simulink model "system_integration_v2"  (R2024a)
settings: Solver=FixedStepDiscrete  StartTime=0.0  StopTime=2  RelTol=1e-3
values from neighbouring files (symbols this model uses):
  Ts = 1/Fs    (= 7.50007500075e-06)    [new_generation_coeff.m]    (also in simon_test.m; simple_fft_test.m = 1/F; testPSD_c2d.m; testPSD_simulink.m)
undefined symbols (not defined in the file or in its folder): magnitude
libraries: hdlsllib x84, embmathops x6, hdlmdlgenlib x1, dsphdlxfrm2 x1
(part 2 of 5)

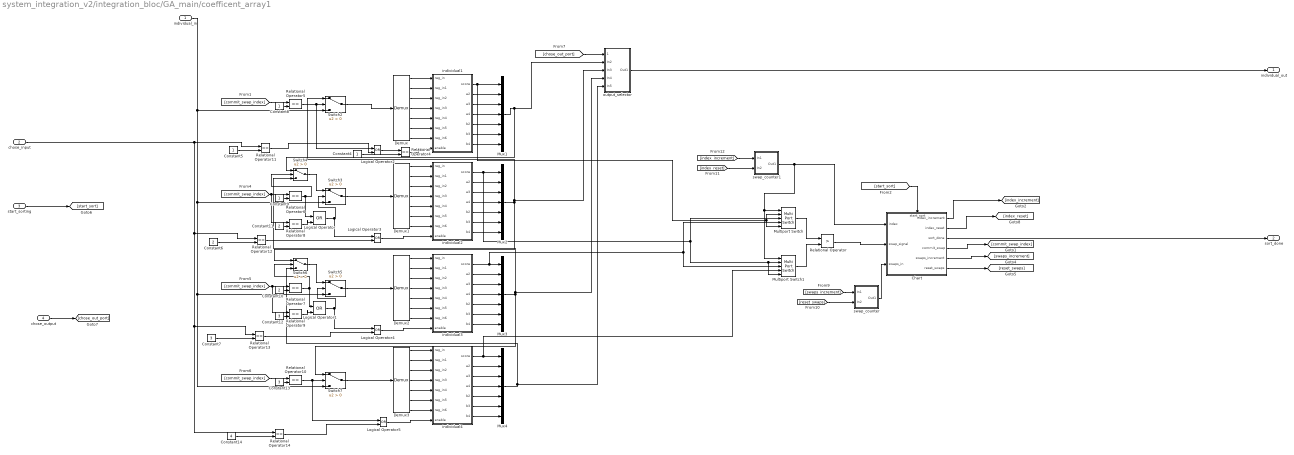
== system system_integration_v2/integration_bloc/GA_main/coefficent_array1 ==
  individual_in : Inport
  chose_input : Inport  Port=2
  start_sorting : Inport  Port=3
  chose_output : Inport  Port=4
  Chart : Stateflow chart  TreatAsAtomicUnit=on
      settings: PortSchema="{\"entries\":[{\"content\":{\"sides\":[{\"content\":{\"connectorIds\":[\"In1\",\"In4\",\"In3\"]},\"type\":\"ConnectorPlacement.EquallySpacedRectSide\",\"uuid\":\"bd2dafac-a5a9-4836-b8bd-cefb36fb6626\"},{\"content\":{\"connectorIds\":[\"Out1\",\"Out2\",\"Out3\",\"Out4\",\"Out5\",\"Out6\"],\"side\":\"RIGHT\"},\"type\":\"ConnectorPlacement.EquallySpacedRectSide\",\"uuid\":\"b2eb894e-8d56-4038-acbe-51c43d919a15\"},{\"content\":{\"connectorIds\":[\"In2\"],\"side\":\"TOP\"},\"type\":\"ConnectorPlacement.EquallySpacedRectSide\",\"uuid\":\"645ecb99-1eca-4a2d-8e44-d34ac75e3d1a\"}]},\"type\":\"ConnectorPlacement.EquallySpacedConnector\",\"uuid\":\"63f53eab-c5ec-482c-b992-d953653b0c27\"}],\"packageUris\":[\"http://schema.mathworks.com/mf0/Connector/R2020b\"],\"version\":\"1.0\"}"
  Constant10 : Constant  Value=2  OutDataTypeStr=fixdt(0,4,0)  SampleTime=Ts
  Constant11 : Constant  Value=2  OutDataTypeStr=fixdt(0,4,0)  SampleTime=Ts
  Constant12 : Constant  Value=3  OutDataTypeStr=fixdt(0,4,0)  SampleTime=Ts
  Constant13 : Constant  Value=3  OutDataTypeStr=fixdt(0,4,0)  SampleTime=Ts
  Constant14 : Constant  Value=4  OutDataTypeStr=fixdt(0,4,0)  SampleTime=Ts
  Constant{4..5,8..9} (4 alike) : Constant  OutDataTypeStr=fixdt(0,4,0)  SampleTime=Ts
  Constant6 : Constant  Value=2  OutDataTypeStr=fixdt(0,4,0)  SampleTime=Ts
  Constant7 : Constant  Value=3  OutDataTypeStr=fixdt(0,4,0)  SampleTime=Ts
  Demux{,1..3} (4 alike) : Demux  Outputs=7
  Logical Operator{,1..5} (6 alike) : Logic  Operator=OR  IconShape=distinctive  AllPortsSameDT=off  OutDataTypeStr=boolean
  Multiport Switch : MultiPortSwitch  DataPortForDefault=Additional data port  DiagnosticForDefault=None  SaturateOnIntegerOverflow=off  InputSameDT=off
  Multiport Switch1 : MultiPortSwitch  DataPortForDefault=Additional data port  DiagnosticForDefault=None  SaturateOnIntegerOverflow=off  InputSameDT=off
  Mux{1..4} (4 alike) : Mux  Inputs=7
  Relational Operator : RelationalOperator  Operator=>  OutDataTypeStr=boolean  InputSameDT=off
  Relational Operator{4..14} (11 alike) : RelationalOperator  Operator===  OutDataTypeStr=boolean  RndMeth=Simplest  InputSameDT=off
  Switch{2..7} (6 alike) : Switch  Criteria=u2 > Threshold  SaturateOnIntegerOverflow=off  InputSameDT=off
  individual1 : Subsystem
  individual2 : Subsystem
  individual3 : Subsystem
  individual4 : Subsystem
  output_selector : Subsystem
  swap_counter : Subsystem
  swap_counter1 : Subsystem
  individual_out : Outport  OutDataTypeStr=fixdt(1,64,32)
  sort_done : Outport  Port=2
  wires:
  individual4/7(b4) -> Mux4/7
  individual4/6(b3) -> Mux4/6
  individual4/5(b2) -> Mux4/5
  individual4/4(a4) -> Mux4/4
  individual4/3(a3) -> Mux4/3
  individual4/2(a2) -> Mux4/2
  Demux3/7 -> individual4/7(reg_in6)
  Demux3/6 -> individual4/6(reg_in5)
  Demux3/5 -> individual4/5(reg_in4)
  Demux3/4 -> individual4/4(reg_in3)
  Demux3/3 -> individual4/3(reg_in2)
  Demux3/2 -> individual4/2(reg_in1)
  Demux3/1 -> individual4/1(reg_in)
  individual3/7(b4) -> Mux3/7
  individual3/6(b3) -> Mux3/6
  individual3/5(b2) -> Mux3/5
  individual3/4(a4) -> Mux3/4
  individual3/3(a3) -> Mux3/3
  individual3/2(a2) -> Mux3/2
  Demux2/7 -> individual3/7(reg_in6)
  Demux2/6 -> individual3/6(reg_in5)
  Demux2/5 -> individual3/5(reg_in4)
  Demux2/4 -> individual3/4(reg_in3)
  Demux2/3 -> individual3/3(reg_in2)
  Demux2/2 -> individual3/2(reg_in1)
  Demux2/1 -> individual3/1(reg_in)
  Demux1/6 -> individual2/6(reg_in5)
  Demux1/5 -> individual2/5(reg_in4)
  Demux1/4 -> individual2/4(reg_in3)
  Demux1/3 -> individual2/3(reg_in2)
  Demux1/2 -> individual2/2(reg_in1)
  Demux1/1 -> individual2/1(reg_in)
  Demux1/7 -> individual2/7(reg_in6)
  individual2/7(b4) -> Mux2/7
  individual2/6(b3) -> Mux2/6
  individual2/5(b2) -> Mux2/5
  individual2/4(a4) -> Mux2/4
  individual1/7(b4) -> Mux1/7
  Demux/7 -> individual1/7(reg_in6)
  Mux4/1 -> output_selector/5(In5), Switch6/3
  Chart/2(index_reset) -> [index_reset]
  [index_reset] -> swap_counter1/2(In2)
  [index_increment] -> swap_counter1/1(In1)
  Constant14/1 -> Relational Operator14/2
  Relational Operator14/1 -> Logical Operator5/2
  Relational Operator13/1 -> Logical Operator4/2
  Constant7/1 -> Relational Operator13/2
  Relational Operator12/1 -> Logical Operator3/2
  Constant6/1 -> Relational Operator12/2
  Relational Operator11/1 -> Logical Operator2/2
  Constant5/1 -> Relational Operator11/2
  chose_output/1 -> [chose_out_port]
  Chart/3(sort_done) -> sort_done/1
  [start_sort] -> Chart/2(start_sort)
  individual2/3(a3) -> Mux2/3
  individual1/4(a4) -> Mux1/4
  Demux/4 -> individual1/4(reg_in3)
  individual1/2(a2) -> Mux1/2
  Relational Operator4/1 -> individual1/8(enable)
  individual1/6(b3) -> Mux1/6
  Demux/2 -> individual1/2(reg_in1)
  individual1/5(b2) -> Mux1/5
  Logical Operator2/1 -> Relational Operator4/1
  Constant10/1 -> Relational Operator7/2
  Relational Operator9/1 -> Logical Operator1/2
  Switch2/1 -> Demux/1
  Multiport Switch1/1 -> Relational Operator/2
  Relational Operator7/1 -> Switch6/2, Logical Operator1/1
  individual2/2(a2) -> Mux2/2
  Switch5/1 -> Demux2/1
  Chart/1(index_increment) -> [index_increment]
  Switch7/1 -> Demux3/1
  Constant8/1 -> Relational Operator5/2
  individual3/1(score) -> Multiport Switch/4, Multiport Switch1/3, Mux3/1
  Mux2/1 -> Switch6/1, Switch2/1, output_selector/3(In3)
  Demux/3 -> individual1/3(reg_in2)
  Logical Operator4/1 -> individual3/8(enable)
  Relational Operator/1 -> Chart/4(swap_signal)
  chose_input/1 -> Relational Operator11/1, Relational Operator12/1, Relational Operator13/1, Relational Operator14/1
  Demux/6 -> individual1/6(reg_in5)
  [chose_out_port] -> output_selector/1(chose_port)
  individual2/1(score) -> Multiport Switch1/2, Multiport Switch1/5, Multiport Switch/3, Mux2/1
  output_selector/1(Out1) -> individual_out/1
  Switch6/1 -> Switch5/1
  [commit_swap_index] -> Relational Operator10/1
  Constant12/1 -> Relational Operator9/2
  Constant13/1 -> Relational Operator10/2
  Constant4/1 -> Relational Operator4/2
  Relational Operator6/1 -> Switch4/2, Logical Operator/1
  individual4/1(score) -> Mux4/1, Multiport Switch1/4
  Switch3/1 -> Demux1/1
  individual_in/1 -> Switch2/3, Switch3/3, Switch5/3, Switch7/3
  Demux/5 -> individual1/5(reg_in4)
  Logical Operator/1 -> Switch3/2, Logical Operator3/1
  Chart/4(commit_swap) -> [commit_swap_index]
  start_sorting/1 -> [start_sort]
  Constant11/1 -> Relational Operator8/2
  Multiport Switch/1 -> Relational Operator/1
  Logical Operator5/1 -> individual4/8(enable)
  Logical Operator3/1 -> individual2/8(enable)
  [commit_swap_index] -> Relational Operator7/1, Relational Operator9/1
  [commit_swap_index] -> Relational Operator6/1, Relational Operator8/1
  Relational Operator8/1 -> Logical Operator/2
  Chart/6(reset_swaps) -> [reset_swaps]
  Mux1/1 -> output_selector/2(In2), Switch4/1
  [commit_swap_index] -> Relational Operator5/1
  [swaps_increment] -> swap_counter/1(In1)
  Relational Operator5/1 -> Switch2/2, Logical Operator2/1
  individual1/3(a3) -> Mux1/3
  swap_counter/1(Out1) -> Chart/3(swaps_in)
  [reset_swaps] -> swap_counter/2(In2)
  Relational Operator10/1 -> Switch7/2, Logical Operator5/1
  Mux3/1 -> Switch7/1, Switch4/3, output_selector/4(In4)
  Demux/1 -> individual1/1(reg_in)
  individual1/1(score) -> Multiport Switch/2, Multiport Switch/5, Mux1/1
  Switch4/1 -> Switch3/1
  swap_counter1/1(Out1) -> Chart/1(index), Multiport Switch/1, Multiport Switch1/1
  Chart/5(swaps_increment) -> [swaps_increment]
  Constant9/1 -> Relational Operator6/2
  Logical Operator1/1 -> Switch5/2, Logical Operator4/1

== system system_integration_v2/integration_bloc/GA_main/generation_counter ==
  In1 : Inport
  In2 : Inport  Port=2
  Add : Sum  OutDataTypeStr=fixdt(0,16,0)  AccumDataTypeStr=fixdt(0,16,0)
  Constant18 : Constant  OutDataTypeStr=fixdt(0,16,0)  SampleTime=Ts
  Constant19 : Constant  Value=0  OutDataTypeStr=fixdt(0,16,0)  SampleTime=Ts
  Constant20 : Constant  Value=0  OutDataTypeStr=fixdt(0,16,0)  SampleTime=Ts
  Delay : Delay  DelayLength=1  InitialCondition=0  SampleTime=Ts
  Switch : Switch  Criteria=u2 > Threshold  OutDataTypeStr=fixdt(0,16,0)  SaturateOnIntegerOverflow=off  InputSameDT=off
  Switch8 : Switch  Criteria=u2 > Threshold  OutDataTypeStr=fixdt(0,16,0)  SaturateOnIntegerOverflow=off  InputSameDT=off
  Out1 : Outport
  wires:
  Constant19/1 -> Switch/3
  Switch8/1 -> Add/2
  Switch/1 -> Add/1
  Delay/1 -> Out1/1, Switch8/3
  In2/1 -> Switch8/2
  Add/1 -> Delay/1
  Constant20/1 -> Switch8/1
  Constant18/1 -> Switch/1
  In1/1 -> Switch/2

== system system_integration_v2/integration_bloc/GA_main/index_counter ==
  In1 : Inport
  In2 : Inport  Port=2
  Add : Sum  OutDataTypeStr=fixdt(0,4,0)  AccumDataTypeStr=fixdt(0,4,0)
  Constant18 : Constant  OutDataTypeStr=fixdt(0,4,0)  SampleTime=Ts
  Constant19 : Constant  Value=0  OutDataTypeStr=fixdt(0,4,0)  SampleTime=Ts
  Constant20 : Constant  Value=0  OutDataTypeStr=fixdt(0,4,0)  SampleTime=Ts
  Delay : Delay  DelayLength=1  InitialCondition=0  SampleTime=Ts
  Switch : Switch  Criteria=u2 > Threshold  OutDataTypeStr=fixdt(0,4,0)  SaturateOnIntegerOverflow=off  InputSameDT=off
  Switch8 : Switch  Criteria=u2 > Threshold  OutDataTypeStr=fixdt(0,4,0)  SaturateOnIntegerOverflow=off  InputSameDT=off
  index_counter : Outport
  wires:
  Constant19/1 -> Switch/3
  Switch8/1 -> Add/2
  Switch/1 -> Add/1
  Delay/1 -> index_counter/1, Switch8/3
  In2/1 -> Switch8/2
  Add/1 -> Delay/1
  Constant20/1 -> Switch8/1
  Constant18/1 -> Switch/1
  In1/1 -> Switch/2

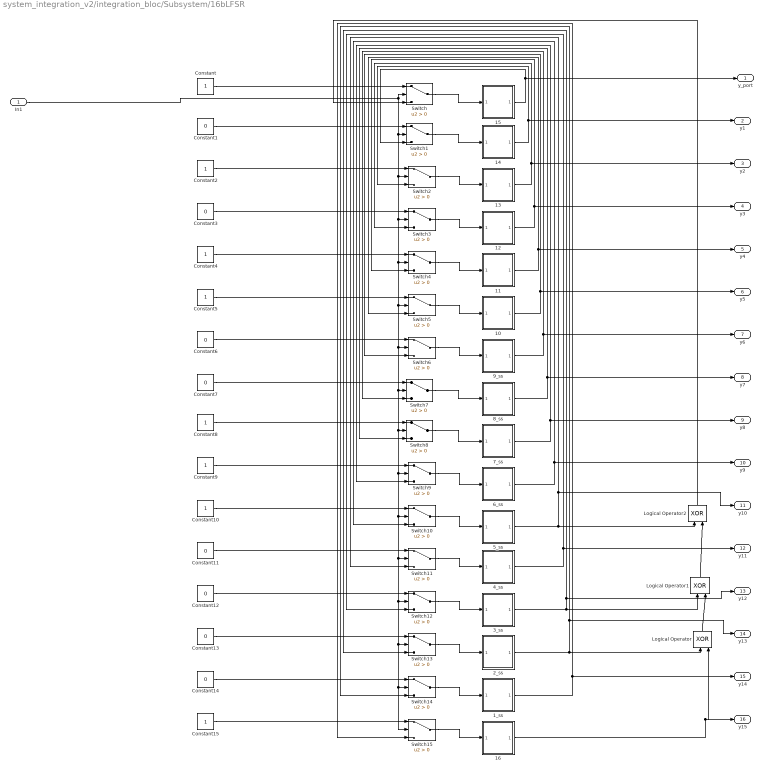
== system system_integration_v2/integration_bloc/Subsystem/16bLFSR ==
  In1 : Inport
  10 : Subsystem
  11 : Subsystem
  12 : Subsystem
  13 : Subsystem
  14 : Subsystem
  15 : Subsystem
  16 : Subsystem
  1_ss : Subsystem
  2_ss : Subsystem
  3_ss : Subsystem
  4_ss : Subsystem
  5_ss : Subsystem
  6_ss : Subsystem
  7_ss : Subsystem
  8_ss : Subsystem
  9_ss : Subsystem
  Constant{,2,4..5,8..10,15} (8 alike) : Constant  OutDataTypeStr=boolean  SampleTime=Ts
  Constant{1,3,6..7,11..14} (8 alike) : Constant  Value=0  OutDataTypeStr=boolean  SampleTime=Ts
  Logical Operator : Logic  Operator=XOR  IconShape=distinctive  AllPortsSameDT=off  OutDataTypeStr=boolean
  Logical Operator1 : Logic  Operator=XOR  IconShape=distinctive  AllPortsSameDT=off  OutDataTypeStr=boolean
  Logical Operator2 : Logic  Operator=XOR  IconShape=distinctive  AllPortsSameDT=off  OutDataTypeStr=boolean
  Switch{,1..15} (16 alike) : Switch  Criteria=u2 > Threshold  SaturateOnIntegerOverflow=off  InputSameDT=off
  y_port : Outport
  y1 : Outport  Port=2
  y2 : Outport  Port=3
  y3 : Outport  Port=4
  y4 : Outport  Port=5
  y5 : Outport  Port=6
  y6 : Outport  Port=7
  y7 : Outport  Port=8
  y8 : Outport  Port=9
  y9 : Outport  Port=10
  y10 : Outport  Port=11
  y11 : Outport  Port=12
  y12 : Outport  Port=13
  y13 : Outport  Port=14
  y14 : Outport  Port=15
  y15 : Outport  Port=16
  wires:
  5_ss/1(reg_out) -> Logical Operator2/1, y10/1, Switch11/3
  6_ss/1(reg_out) -> y9/1, Switch10/3
  2_ss/1(reg_out) -> Logical Operator/1, y13/1, Switch14/3
  11/1(reg_out) -> y4/1, Switch5/3
  Logical Operator2/1 -> Switch/3
  Constant13/1 -> Switch13/1
  Switch13/1 -> 2_ss/1(reg_in)
  3_ss/1(reg_out) -> Logical Operator1/1, y12/1, Switch13/3
  4_ss/1(reg_out) -> y11/1, Switch12/3
  Constant/1 -> Switch/1
  Constant4/1 -> Switch4/1
  Constant2/1 -> Switch2/1
  In1/1 -> Switch/2, Switch15/2, Switch14/2, Switch13/2, Switch12/2, Switch11/2, Switch10/2, Switch9/2, Switch8/2, Switch7/2, Switch6/2, Switch5/2, Switch4/2, Switch3/2, Switch2/2, Switch1/2
  Switch12/1 -> 3_ss/1(reg_in)
  15/1(reg_out) -> y_port/1, Switch1/3
  Switch1/1 -> 14/1(reg_in)
  Constant8/1 -> Switch8/1
  Constant6/1 -> Switch6/1
  Constant5/1 -> Switch5/1
  Constant14/1 -> Switch14/1
  Constant11/1 -> Switch11/1
  Switch5/1 -> 10/1(reg_in)
  Constant9/1 -> Switch9/1
  Logical Operator/1 -> Logical Operator1/2
  Switch2/1 -> 13/1(reg_in)
  7_ss/1(reg_out) -> y8/1, Switch9/3
  Logical Operator1/1 -> Logical Operator2/2
  Switch11/1 -> 4_ss/1(reg_in)
  Constant7/1 -> Switch7/1
  Switch6/1 -> 9_ss/1(reg_in)
  Switch/1 -> 15/1(reg_in)
  Constant12/1 -> Switch12/1
  Switch4/1 -> 11/1(reg_in)
  Constant15/1 -> Switch15/1
  16/1(reg_out) -> y15/1, Logical Operator/2
  13/1(reg_out) -> y2/1, Switch3/3
  Switch9/1 -> 6_ss/1(reg_in)
  Switch7/1 -> 8_ss/1(reg_in)
  Constant10/1 -> Switch10/1
  Switch14/1 -> 1_ss/1(reg_in)
  Switch3/1 -> 12/1(reg_in)
  Switch15/1 -> 16/1(reg_in)
  9_ss/1(reg_out) -> y6/1, Switch7/3
  Constant3/1 -> Switch3/1
  Constant1/1 -> Switch1/1
  14/1(reg_out) -> y1/1, Switch2/3
  Switch10/1 -> 5_ss/1(reg_in)
  10/1(reg_out) -> y5/1, Switch6/3
  Switch8/1 -> 7_ss/1(reg_in)
  12/1(reg_out) -> y3/1, Switch4/3
  8_ss/1(reg_out) -> y7/1, Switch8/3
  1_ss/1(reg_out) -> y14/1, Switch15/3

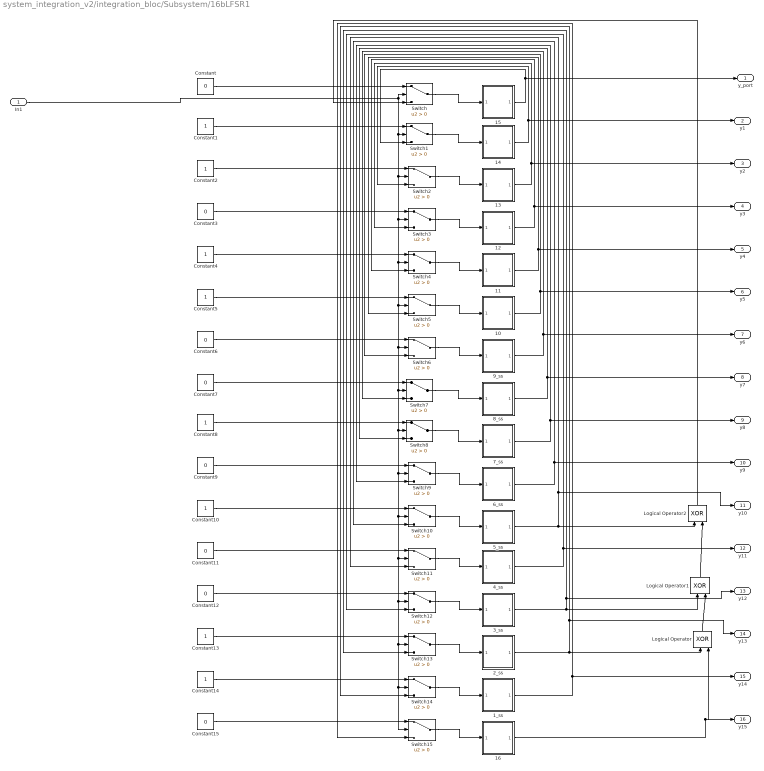
== system system_integration_v2/integration_bloc/Subsystem/16bLFSR1 ==
  In1 : Inport
  10 : Subsystem
  11 : Subsystem
  12 : Subsystem
  13 : Subsystem
  14 : Subsystem
  15 : Subsystem
  16 : Subsystem
  1_ss : Subsystem
  2_ss : Subsystem
  3_ss : Subsystem
  4_ss : Subsystem
  5_ss : Subsystem
  6_ss : Subsystem
  7_ss : Subsystem
  8_ss : Subsystem
  9_ss : Subsystem
  Constant{,3,6..7,9,11..12,15} (8 alike) : Constant  Value=0  OutDataTypeStr=boolean  SampleTime=Ts
  Constant{1..2,4..5,8,10,13..14} (8 alike) : Constant  OutDataTypeStr=boolean  SampleTime=Ts
  Logical Operator : Logic  Operator=XOR  IconShape=distinctive  AllPortsSameDT=off  OutDataTypeStr=boolean
  Logical Operator1 : Logic  Operator=XOR  IconShape=distinctive  AllPortsSameDT=off  OutDataTypeStr=boolean
  Logical Operator2 : Logic  Operator=XOR  IconShape=distinctive  AllPortsSameDT=off  OutDataTypeStr=boolean
  Switch{,1..15} (16 alike) : Switch  Criteria=u2 > Threshold  SaturateOnIntegerOverflow=off  InputSameDT=off
  y_port : Outport
  y1 : Outport  Port=2
  y2 : Outport  Port=3
  y3 : Outport  Port=4
  y4 : Outport  Port=5
  y5 : Outport  Port=6
  y6 : Outport  Port=7
  y7 : Outport  Port=8
  y8 : Outport  Port=9
  y9 : Outport  Port=10
  y10 : Outport  Port=11
  y11 : Outport  Port=12
  y12 : Outport  Port=13
  y13 : Outport  Port=14
  y14 : Outport  Port=15
  y15 : Outport  Port=16
  wires:
  1_ss/1(reg_out) -> Switch15/3, y14/1
  8_ss/1(reg_out) -> Switch8/3, y7/1
  12/1(reg_out) -> Switch4/3, y3/1
  Switch8/1 -> 7_ss/1(reg_in)
  10/1(reg_out) -> Switch6/3, y5/1
  Switch10/1 -> 5_ss/1(reg_in)
  14/1(reg_out) -> Switch2/3, y1/1
  Constant1/1 -> Switch1/1
  Constant3/1 -> Switch3/1
  9_ss/1(reg_out) -> Switch7/3, y6/1
  Switch15/1 -> 16/1(reg_in)
  Switch3/1 -> 12/1(reg_in)
  Switch14/1 -> 1_ss/1(reg_in)
  Constant10/1 -> Switch10/1
  Switch7/1 -> 8_ss/1(reg_in)
  Switch9/1 -> 6_ss/1(reg_in)
  13/1(reg_out) -> Switch3/3, y2/1
  16/1(reg_out) -> Logical Operator/2, y15/1
  Constant15/1 -> Switch15/1
  Switch4/1 -> 11/1(reg_in)
  Constant12/1 -> Switch12/1
  Switch/1 -> 15/1(reg_in)
  Switch6/1 -> 9_ss/1(reg_in)
  Constant7/1 -> Switch7/1
  Switch11/1 -> 4_ss/1(reg_in)
  Logical Operator1/1 -> Logical Operator2/2
  7_ss/1(reg_out) -> Switch9/3, y8/1
  Switch2/1 -> 13/1(reg_in)
  Logical Operator/1 -> Logical Operator1/2
  Constant9/1 -> Switch9/1
  Switch5/1 -> 10/1(reg_in)
  Constant11/1 -> Switch11/1
  Constant14/1 -> Switch14/1
  Constant5/1 -> Switch5/1
  Constant6/1 -> Switch6/1
  Constant8/1 -> Switch8/1
  Switch1/1 -> 14/1(reg_in)
  15/1(reg_out) -> Switch1/3, y_port/1
  Switch12/1 -> 3_ss/1(reg_in)
  In1/1 -> Switch1/2, Switch2/2, Switch3/2, Switch4/2, Switch5/2, Switch6/2, Switch7/2, Switch8/2, Switch9/2, Switch10/2, Switch11/2, Switch12/2, Switch13/2, Switch14/2, Switch15/2, Switch/2
  Constant2/1 -> Switch2/1
  Constant4/1 -> Switch4/1
  Constant/1 -> Switch/1
  4_ss/1(reg_out) -> Switch12/3, y11/1
  3_ss/1(reg_out) -> Switch13/3, y12/1, Logical Operator1/1
  Switch13/1 -> 2_ss/1(reg_in)
  Constant13/1 -> Switch13/1
  Logical Operator2/1 -> Switch/3
  11/1(reg_out) -> Switch5/3, y4/1
  2_ss/1(reg_out) -> Switch14/3, y13/1, Logical Operator/1
  6_ss/1(reg_out) -> Switch10/3, y9/1
  5_ss/1(reg_out) -> Switch11/3, y10/1, Logical Operator2/1

== system system_integration_v2/integration_bloc/Subsystem/a2_random ==
  In1 : Inport
  In2 : Inport  Port=2
  Add : Sum  Inputs=+-  OutDataTypeStr=Inherit: Same as first input
  Add1 : Sum  OutDataTypeStr=Inherit: Same as first input
  Bit Shift : hdlsllib/Logic and Bit Operations/Bit Shift  mode=Shift Right Logical  N=16+5
  Constant : Constant  OutDataTypeStr=boolean  SampleTime=Ts
  Constant16 : Constant  Value=-1.975  OutDataTypeStr=fixdt(1,17,15)  SampleTime=Ts
  Data Type Conversion : DataTypeConversion  OutDataTypeStr=fixdt(0,11,11)  SaturateOnIntegerOverflow=off  RndMeth=Floor
  Data Type Conversion1 : DataTypeConversion  OutDataTypeStr=fixdt(0,32,16)  SaturateOnIntegerOverflow=off  RndMeth=Floor
  Data Type Conversion2 : DataTypeConversion  OutDataTypeStr=fixdt(1,17,15)  SaturateOnIntegerOverflow=off  RndMeth=Floor
  Modulo by Constant HDL Optimized1 : embmathops/Modulo by Constant HDL Optimized  Denominator=0.025  SimulateUsing=Code generation
      settings: LibrarySourceBlock=|
      | embeddedMatrixLib/Math Operations/Modulo by Constant
      | HDL Optimized
  Scope{1..5} (5 alike) : Scope
  Switch16 : Switch  Criteria=u2 > Threshold  SaturateOnIntegerOverflow=off  InputSameDT=off
  Terminator : Terminator
  Out1 : Outport
  wires:
  Data Type Conversion2/1 -> Add/2, Add1/1
  Bit Shift/1 -> Scope4/1, Data Type Conversion/1
  Add1/1 -> Switch16/3
  Add/1 -> Switch16/1
  Data Type Conversion1/1 -> Scope3/1, Bit Shift/1
  Constant16/1 -> Add1/2, Add/1
  Switch16/1 -> Scope1/1, Out1/1
  Data Type Conversion/1 -> Modulo by Constant HDL Optimized1/1, Scope5/1
  In2/1 -> Switch16/2
  In1/1 -> Scope2/1, Data Type Conversion1/1
  Constant/1 -> Modulo by Constant HDL Optimized1/2
  Modulo by Constant HDL Optimized1/2 -> Terminator/1
  Modulo by Constant HDL Optimized1/1 -> Data Type Conversion2/1

== system system_integration_v2/integration_bloc/Subsystem/a3_random ==
  In1 : Inport
  In2 : Inport  Port=2
  Add6 : Sum  Inputs=+-  OutDataTypeStr=Inherit: Same as first input
  Add7 : Sum  OutDataTypeStr=Inherit: Same as first input
  Bit Shift3 : hdlsllib/Logic and Bit Operations/Bit Shift  mode=Shift Right Logical  N=16+6
  Constant : Constant  OutDataTypeStr=boolean  SampleTime=Ts
  Constant3 : Constant  Value=1.0286  OutDataTypeStr=fixdt(1,18,15)  SampleTime=Ts
  Data Type Conversion10 : DataTypeConversion  OutDataTypeStr=fixdt(0,32,16)  SaturateOnIntegerOverflow=off  RndMeth=Floor
  Data Type Conversion11 : DataTypeConversion  OutDataTypeStr=fixdt(1,18,15)  SaturateOnIntegerOverflow=off  RndMeth=Floor
  Data Type Conversion9 : DataTypeConversion  OutDataTypeStr=fixdt(0,11,11)  SaturateOnIntegerOverflow=off  RndMeth=Floor
  Modulo by Constant HDL Optimized : embmathops/Modulo by Constant HDL Optimized  Denominator=0.0106  SimulateUsing=Code generation
      settings: LibrarySourceBlock=|
      | embeddedMatrixLib/Math Operations/Modulo by Constant
      | HDL Optimized
  Scope{2..5} (4 alike) : Scope
  Switch3 : Switch  Criteria=u2 > Threshold  SaturateOnIntegerOverflow=off  InputSameDT=off
  Terminator : Terminator
  Out1 : Outport
  wires:
  Constant3/1 -> Add6/1, Add7/2
  Modulo by Constant HDL Optimized/1 -> Data Type Conversion11/1
  Add6/1 -> Switch3/1
  Data Type Conversion11/1 -> Add7/1, Add6/2
  Add7/1 -> Switch3/3
  In2/1 -> Switch3/2
  Switch3/1 -> Out1/1
  In1/1 -> Scope2/1, Data Type Conversion10/1
  Bit Shift3/1 -> Scope4/1, Data Type Conversion9/1
  Data Type Conversion9/1 -> Modulo by Constant HDL Optimized/1, Scope5/1
  Data Type Conversion10/1 -> Scope3/1, Bit Shift3/1
  Constant/1 -> Modulo by Constant HDL Optimized/2
  Modulo by Constant HDL Optimized/2 -> Terminator/1

== system system_integration_v2/integration_bloc/Subsystem/a4_random ==
  In1 : Inport
  In2 : Inport  Port=2
  Add4 : Sum  Inputs=+-  OutDataTypeStr=Inherit: Same as first input
  Add5 : Sum  OutDataTypeStr=Inherit: Same as first input
  Bit Shift2 : hdlsllib/Logic and Bit Operations/Bit Shift  mode=Shift Right Logical  N=16+6
  Constant : Constant  OutDataTypeStr=boolean  SampleTime=Ts
  Constant2 : Constant  Value=-0.04  OutDataTypeStr=fixdt(1,17,15)  SampleTime=Ts
  Data Type Conversion6 : DataTypeConversion  OutDataTypeStr=fixdt(0,11,11)  SaturateOnIntegerOverflow=off  RndMeth=Floor
  Data Type Conversion7 : DataTypeConversion  OutDataTypeStr=fixdt(0,32,16)  SaturateOnIntegerOverflow=off  RndMeth=Floor
  Data Type Conversion8 : DataTypeConversion  OutDataTypeStr=fixdt(1,17,15)  SaturateOnIntegerOverflow=off  RndMeth=Floor
  Modulo by Constant HDL Optimized : embmathops/Modulo by Constant HDL Optimized  Denominator=0.008  SimulateUsing=Code generation
      settings: LibrarySourceBlock=|
      | embeddedMatrixLib/Math Operations/Modulo by Constant
      | HDL Optimized
  Scope{2..5} (4 alike) : Scope
  Switch2 : Switch  Criteria=u2 > Threshold  SaturateOnIntegerOverflow=off  InputSameDT=off
  Terminator : Terminator
  Out1 : Outport
  wires:
  Data Type Conversion8/1 -> Add4/2, Add5/1
  Modulo by Constant HDL Optimized/1 -> Data Type Conversion8/1
  Constant2/1 -> Add5/2, Add4/1
  In2/1 -> Switch2/2
  Add4/1 -> Switch2/1
  Add5/1 -> Switch2/3
  Switch2/1 -> Out1/1
  In1/1 -> Scope2/1, Data Type Conversion7/1
  Bit Shift2/1 -> Scope4/1, Data Type Conversion6/1
  Data Type Conversion6/1 -> Modulo by Constant HDL Optimized/1, Scope5/1
  Data Type Conversion7/1 -> Scope3/1, Bit Shift2/1
  Constant/1 -> Modulo by Constant HDL Optimized/2
  Modulo by Constant HDL Optimized/2 -> Terminator/1

== system system_integration_v2/integration_bloc/Subsystem/b2_random ==
  In1 : Inport
  In2 : Inport  Port=2
  Add6 : Sum  Inputs=+-  OutDataTypeStr=Inherit: Same as first input
  Add7 : Sum  OutDataTypeStr=Inherit: Same as first input
  Bit Shift3 : hdlsllib/Logic and Bit Operations/Bit Shift  mode=Shift Right Logical  N=16+6
  Constant : Constant  OutDataTypeStr=boolean  SampleTime=Ts
  Constant3 : Constant  Value=-1.9970  OutDataTypeStr=fixdt(1,18,15)  SampleTime=Ts
  Data Type Conversion10 : DataTypeConversion  OutDataTypeStr=fixdt(0,32,16)  SaturateOnIntegerOverflow=off  RndMeth=Floor
  Data Type Conversion11 : DataTypeConversion  OutDataTypeStr=fixdt(1,18,15)  SaturateOnIntegerOverflow=off  RndMeth=Floor
  Data Type Conversion9 : DataTypeConversion  OutDataTypeStr=fixdt(0,11,11)  RndMeth=Floor
  Modulo by Constant HDL Optimized : embmathops/Modulo by Constant HDL Optimized  Denominator=0.0130  SimulateUsing=Code generation
      settings: LibrarySourceBlock=|
      | embeddedMatrixLib/Math Operations/Modulo by Constant
      | HDL Optimized
  Switch3 : Switch  Criteria=u2 > Threshold  SaturateOnIntegerOverflow=off  InputSameDT=off
  Terminator : Terminator
  Out1 : Outport
  wires:
  Constant3/1 -> Add6/1, Add7/2
  Modulo by Constant HDL Optimized/1 -> Data Type Conversion11/1
  Add6/1 -> Switch3/1
  Data Type Conversion11/1 -> Add7/1, Add6/2
  Add7/1 -> Switch3/3
  In2/1 -> Switch3/2
  Switch3/1 -> Out1/1
  In1/1 -> Data Type Conversion10/1
  Bit Shift3/1 -> Data Type Conversion9/1
  Data Type Conversion9/1 -> Modulo by Constant HDL Optimized/1
  Data Type Conversion10/1 -> Bit Shift3/1
  Constant/1 -> Modulo by Constant HDL Optimized/2
  Modulo by Constant HDL Optimized/2 -> Terminator/1

== system system_integration_v2/integration_bloc/Subsystem/b3_random ==
  In1 : Inport
  In2 : Inport  Port=2
  Add6 : Sum  Inputs=+-  OutDataTypeStr=Inherit: Same as first input
  Add7 : Sum  OutDataTypeStr=Inherit: Same as first input
  Bit Shift3 : hdlsllib/Logic and Bit Operations/Bit Shift  mode=Shift Right Logical  N=16+6
  Constant : Constant  OutDataTypeStr=boolean  SampleTime=Ts
  Constant3 : Constant  Value=1.022  OutDataTypeStr=fixdt(1,18,15)  SampleTime=Ts
  Data Type Conversion10 : DataTypeConversion  OutDataTypeStr=fixdt(0,32,16)  SaturateOnIntegerOverflow=off  RndMeth=Floor
  Data Type Conversion11 : DataTypeConversion  OutDataTypeStr=fixdt(1,18,15)  SaturateOnIntegerOverflow=off  RndMeth=Floor
  Data Type Conversion9 : DataTypeConversion  OutDataTypeStr=fixdt(0,11,11)  RndMeth=Floor
  Modulo by Constant HDL Optimized : embmathops/Modulo by Constant HDL Optimized  Denominator=0.01  SimulateUsing=Code generation
      settings: LibrarySourceBlock=|
      | embeddedMatrixLib/Math Operations/Modulo by Constant
      | HDL Optimized
  Scope{2..5} (4 alike) : Scope
  Switch3 : Switch  Criteria=u2 > Threshold  SaturateOnIntegerOverflow=off  InputSameDT=off
  Terminator : Terminator
  Out1 : Outport
  wires:
  Switch3/1 -> Out1/1
  In2/1 -> Switch3/2
  Add7/1 -> Switch3/3
  Data Type Conversion11/1 -> Add6/2, Add7/1
  Add6/1 -> Switch3/1
  Modulo by Constant HDL Optimized/1 -> Data Type Conversion11/1
  Constant3/1 -> Add7/2, Add6/1
  In1/1 -> Scope2/1, Data Type Conversion10/1
  Bit Shift3/1 -> Scope4/1, Data Type Conversion9/1
  Data Type Conversion9/1 -> Modulo by Constant HDL Optimized/1, Scope5/1
  Data Type Conversion10/1 -> Scope3/1, Bit Shift3/1
  Constant/1 -> Modulo by Constant HDL Optimized/2
  Modulo by Constant HDL Optimized/2 -> Terminator/1

== system system_integration_v2/integration_bloc/Subsystem/b4_random ==
  In1 : Inport
  In2 : Inport  Port=2
  Add8 : Sum  Inputs=+-  OutDataTypeStr=Inherit: Same as first input
  Add9 : Sum  OutDataTypeStr=Inherit: Same as first input
  Bit Shift4 : hdlsllib/Logic and Bit Operations/Bit Shift  mode=Shift Right Logical  N=16+12
  Constant : Constant  OutDataTypeStr=boolean  SampleTime=Ts
  Constant4 : Constant  Value=-0.0239  OutDataTypeStr=fixdt(1,18,15)  SampleTime=Ts
  Data Type Conversion12 : DataTypeConversion  OutDataTypeStr=fixdt(0,32,16)  SaturateOnIntegerOverflow=off  RndMeth=Floor
  Data Type Conversion13 : DataTypeConversion  OutDataTypeStr=fixdt(1,18,16)  SaturateOnIntegerOverflow=off  RndMeth=Floor
  Data Type Conversion14 : DataTypeConversion  OutDataTypeStr=fixdt(0,11,11)  SaturateOnIntegerOverflow=off  RndMeth=Floor
  Modulo by Constant HDL Optimized : embmathops/Modulo by Constant HDL Optimized  Denominator=2.5e-4  SimulateUsing=Code generation
      settings: LibrarySourceBlock=|
      | embeddedMatrixLib/Math Operations/Modulo by Constant
      | HDL Optimized
  Scope{1..5} (5 alike) : Scope
  Switch4 : Switch  Criteria=u2 > Threshold  SaturateOnIntegerOverflow=off  InputSameDT=off
  Terminator : Terminator
  Out1 : Outport
  wires:
  Data Type Conversion13/1 -> Add8/2, Add9/1
  Constant4/1 -> Add9/2, Add8/1
  Modulo by Constant HDL Optimized/1 -> Data Type Conversion13/1
  In2/1 -> Switch4/2
  Add9/1 -> Switch4/3
  Add8/1 -> Switch4/1
  Switch4/1 -> Scope1/1, Out1/1
  In1/1 -> Scope2/1, Data Type Conversion12/1
  Bit Shift4/1 -> Scope4/1, Data Type Conversion14/1
  Data Type Conversion14/1 -> Modulo by Constant HDL Optimized/1, Scope5/1
  Data Type Conversion12/1 -> Scope3/1, Bit Shift4/1
  Constant/1 -> Modulo by Constant HDL Optimized/2
  Modulo by Constant HDL Optimized/2 -> Terminator/1

== system system_integration_v2/integration_bloc/Subsystem/random_gene ==
  u1 : Inport
  u2 : Inport  Port=2
  In3 : Inport  Port=3
  In4 : Inport  Port=4
  Add12 : Sum  Inputs=++++  OutDataTypeStr=Inherit: Same as first input
  Constant7 : Constant  OutDataTypeStr=fixdt(0,3,0)  SampleTime=Ts
  Data Type Conversion17 : DataTypeConversion  OutDataTypeStr=fixdt(0,3,0)  SaturateOnIntegerOverflow=off  RndMeth=Floor
  Data Type Conversion18 : DataTypeConversion  OutDataTypeStr=fixdt(0,3,0)  SaturateOnIntegerOverflow=off  RndMeth=Floor
  Data Type Conversion19 : DataTypeConversion  OutDataTypeStr=fixdt(0,3,0)  SaturateOnIntegerOverflow=off  RndMeth=Floor
  concat3 : hdlsllib/Logic and Bit Operations/Bit Concat  numInputs=2
  Out1 : Outport
  wires:
  In3/1 -> Data Type Conversion18/1
  Data Type Conversion18/1 -> Add12/2
  u1/1 -> concat3/1
  u2/1 -> concat3/2
  Add12/1 -> Out1/1
  Data Type Conversion17/1 -> Add12/4
  concat3/1 -> Data Type Conversion17/1
  Constant7/1 -> Add12/3
  Data Type Conversion19/1 -> Add12/1
  In4/1 -> Data Type Conversion19/1

== system system_integration_v2/integration_bloc/Subsystem/random_method ==
  u1 : Inport
  u2 : Inport  Port=2
  Add11 : Sum  OutDataTypeStr=Inherit: Same as first input
  Constant6 : Constant  OutDataTypeStr=fixdt(0,3,0)  SampleTime=Ts
  Data Type Conversion16 : DataTypeConversion  OutDataTypeStr=fixdt(0,3,0)  SaturateOnIntegerOverflow=off  RndMeth=Floor
  concat2 : hdlsllib/Logic and Bit Operations/Bit Concat  numInputs=2
  Out1 : Outport
  wires:
  Constant6/1 -> Add11/2
  Add11/1 -> Out1/1
  concat2/1 -> Data Type Conversion16/1
  u1/1 -> concat2/1
  Data Type Conversion16/1 -> Add11/1
  u2/1 -> concat2/2

== system system_integration_v2/integration_bloc/Subsystem/random_sample ==
  u1 : Inport
  u2 : Inport  Port=2
  Add10 : Sum  OutDataTypeStr=Inherit: Same as first input
  Constant5 : Constant  OutDataTypeStr=fixdt(0,4,0)  SampleTime=Ts
  Data Type Conversion15 : DataTypeConversion  OutDataTypeStr=fixdt(0,4,0)  SaturateOnIntegerOverflow=off  RndMeth=Floor
  concat1 : hdlsllib/Logic and Bit Operations/Bit Concat  numInputs=2
  Out1 : Outport
  wires:
  Add10/1 -> Out1/1
  Constant5/1 -> Add10/2
  Data Type Conversion15/1 -> Add10/1
  concat1/1 -> Data Type Conversion15/1
  u2/1 -> concat1/2
  u1/1 -> concat1/1
